simulink model "CassieRealTimeSubsystem"  (R2016b)
settings: Solver=FixedStepDiscrete  StartTime=0.0  StopTime=inf  RelTol=1e-3  EnableMultiTasking=on
InitFcn:
  | realTimeInitFcn;
undefined symbols (not defined in the file): CassieParameters, leftLegMedulla, pelvisMedulla, rightLegMedulla
libraries: xpcethercatlib x98, RealTimeLibrary x10, slrtlib x4, simulink x3
(part 1 of 2)
settings Model: xpc_rtwmakecfg_data=_xpcethercatlib_  ParamWorkspaceSource=ReferencedWorkspace  Creator=robot  LastModifiedBy=mikha
settings SolverCC: EnableConcurrentExecution=on
settings DataIOCC: SaveFormat=Array  SaveOutput=off  SignalLogging=off  DSMLogging=off  VisualizeSimOutput=off  SaveTime=off
settings OptimizationCC: DefaultParameterBehavior=Inlined  InlineInvariantSignals=on  LifeSpan=inf  SimCompilerOptimization=on  AccelVerboseBuild=on
settings DebuggingCC: AllowSymbolicDim=off  SFUnexpectedBacktrackingDiag=warning  SFNoUnconditionalDefaultTransitionDiag=warning  SFExecutionAtInitializationDiag=none
settings HardwareCC: ProdBitPerPointer=32  ProdBitPerSizeT=32  ProdBitPerPtrDiffT=32  ProdLargestAtomicFloat=None  ProdWordSize=32  ProdLongLongMode=on  ProdHWDeviceType=Generic->32-bit x86 compatible
settings ModelReferenceCC: ParallelModelReferenceMATLABWorkerInit=Copy Base Workspace  ModelReferenceNumInstancesAllowed=Single
settings SFSimCC: SFSimEcho=off
settings RTWCC: SystemTargetFile=slrt.tlc  TLCOptions=-axPCMaxOverloads=1000000000 -axPCMaxOverloadLen=1000000000  TemplateMakefile=slrt_default_tmf  Description=Simulink Real-Time  RTWCompilerOptimization=on
settings CodeAppCC: GenerateComments=off  MaxIdLength=128  SimulinkBlockComments=off
settings SimulinkRealTimeCC: ExtMode=off
settings ConfigComp: CovMetricSettings=dw  CovHtmlReporting=on  CovSaveCumulativeToWorkspaceVar=on  CovSaveSingleToWorkspaceVar=on  CovExternalEMLEnable=off

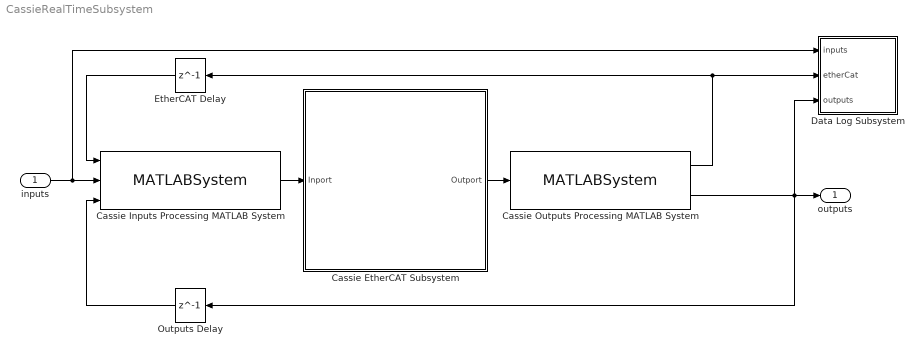
== system CassieRealTimeSubsystem ==
  inputs : Inport  OutDataTypeStr=Bus: cassieInputsBus  PortDimensions=[1 1]  SampleTime=CassieParameters.etherCatSampleTime  BusOutputAsStruct=on
  Cassie EtherCAT Subsystem : Subsystem
      mask Display: image('Cassie.png');
  Cassie Inputs Processing MATLAB System : MATLABSystem  System=ProcessInputs  SimulateUsing=Code generation
      mask Type: ProcessInputs
      mask Display:
      | disp('ProcessInputs');
      | port_label('input',1,'etherCat');
      | port_label('input',2,'inputs');
      | port_label('input',3,'outputs');
      | port_label('output',1,'etherCat');
  Cassie Outputs Processing MATLAB System : MATLABSystem  System=ProcessOutputs  SimulateUsing=Code generation
      mask Type: ProcessOutputs
      mask Display:
      | disp('ProcessOutputs');
      | port_label('input',1,'etherCat');
      | port_label('output',1,'etherCat');
      | port_label('output',2,'outputs');
  Data Log Subsystem : Subsystem
  EtherCAT Delay : Delay  DelayLength=1  InputProcessing=Inherited
  Outputs Delay : Delay  DelayLength=1  InputProcessing=Inherited
  outputs : Outport  OutDataTypeStr=Bus: cassieOutputsBus  PortDimensions=[1 1]  SampleTime=CassieParameters.etherCatSampleTime  BusOutputAsStruct=on
  wires:
  inputs/1 -> Data Log Subsystem/1(inputs), Cassie Inputs Processing MATLAB System/2
  Cassie Outputs Processing MATLAB System/2 -> Data Log Subsystem/3(outputs), Outputs Delay/1, outputs/1
  Cassie EtherCAT Subsystem/1(Outport) -> Cassie Outputs Processing MATLAB System/1
  Cassie Outputs Processing MATLAB System/1 -> EtherCAT Delay/1, Data Log Subsystem/2(etherCat)
  Cassie Inputs Processing MATLAB System/1 -> Cassie EtherCAT Subsystem/1(Inport)
  EtherCAT Delay/1 -> Cassie Inputs Processing MATLAB System/1
  Outputs Delay/1 -> Cassie Inputs Processing MATLAB System/3

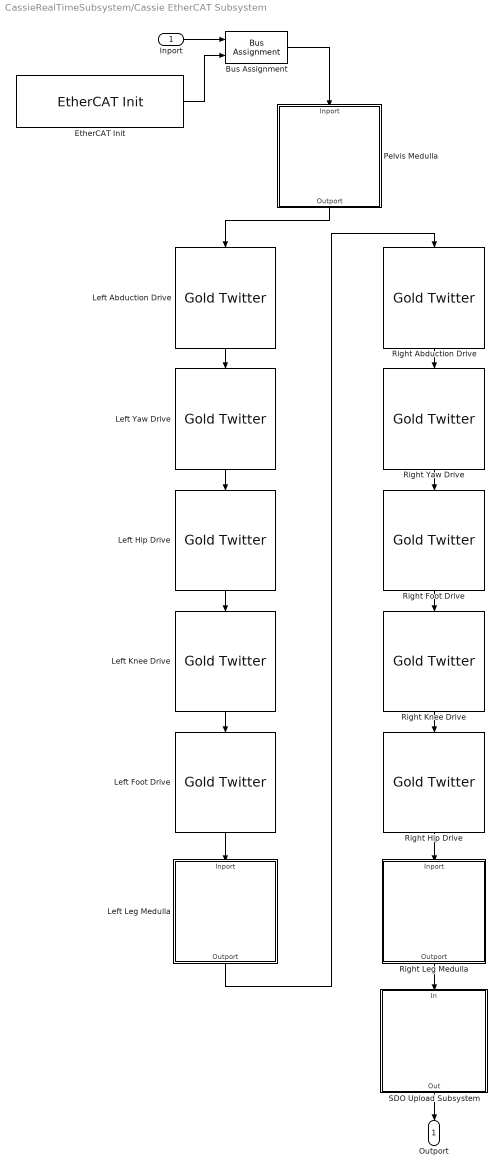
== system CassieRealTimeSubsystem/Cassie EtherCAT Subsystem ==
  Inport : Inport
  Bus Assignment : BusAssignment  AssignedSignals=status
  "EtherCAT Init " : xpcethercatlib/EtherCAT Init   Priority=0  config_file=cassie-v3-eni.xml  device_id=0  pci_bus=CassieParameters.etherCatPciBus  pci_slot=CassieParameters.etherCatPciSlot  dctuning=0  enaDebug=off  enaDC=on  errLink=on  masterDbg=on  stateChgDbg=on  baseClock=on  masterCfg=on  logFile='c:\dbglog2.txt'  sample_time=0.000500  DCMode=1
  Left Abduction Drive : RealTimeLibrary/Gold Twitter  structureName='leftAbductionDrive'  ethercatName='Left Abduction Drive'  gearRatio=CassieParameters.motorGearRatio(1)*CassieParameters.motorDirection(1)  torqueConstant=CassieParameters.motorTorqueConstant(1)  encoderCounts=CassieParameters.motorEncoderTicks(1)  peakCurrentLimit=CassieParameters.twitterPeakCurrent(1)
  Left Foot Drive : RealTimeLibrary/Gold Twitter  structureName='leftFootDrive'  ethercatName='Left Foot Drive'  gearRatio=CassieParameters.motorGearRatio(5)*CassieParameters.motorDirection(5)  torqueConstant=CassieParameters.motorTorqueConstant(5)  encoderCounts=CassieParameters.motorEncoderTicks(5)  peakCurrentLimit=CassieParameters.twitterPeakCurrent(5)
  Left Hip Drive : RealTimeLibrary/Gold Twitter  structureName='leftHipDrive'  ethercatName='Left Hip Drive'  gearRatio=CassieParameters.motorGearRatio(3)*CassieParameters.motorDirection(3)  torqueConstant=CassieParameters.motorTorqueConstant(3)  encoderCounts=CassieParameters.motorEncoderTicks(3)  peakCurrentLimit=CassieParameters.twitterPeakCurrent(3)
  Left Knee Drive : RealTimeLibrary/Gold Twitter  structureName='leftKneeDrive'  ethercatName='Left Knee Drive'  gearRatio=CassieParameters.motorGearRatio(4)*CassieParameters.motorDirection(4)  torqueConstant=CassieParameters.motorTorqueConstant(4)  encoderCounts=CassieParameters.motorEncoderTicks(4)  peakCurrentLimit=CassieParameters.twitterPeakCurrent(4)
  Left Leg Medulla : Subsystem
      mask Display: image('Medulla.png');
  Left Yaw Drive : RealTimeLibrary/Gold Twitter  structureName='leftYawDrive'  ethercatName='Left Yaw Drive'  gearRatio=CassieParameters.motorGearRatio(2)*CassieParameters.motorDirection(2)  torqueConstant=CassieParameters.motorTorqueConstant(2)  encoderCounts=CassieParameters.motorEncoderTicks(2)  peakCurrentLimit=CassieParameters.twitterPeakCurrent(2)
  Pelvis Medulla : Subsystem
      mask Display: image('Medulla.png');
  Right Abduction Drive : RealTimeLibrary/Gold Twitter  structureName='rightAbductionDrive'  ethercatName='Right Abduction Drive'  gearRatio=CassieParameters.motorGearRatio(6)*CassieParameters.motorDirection(6)  torqueConstant=CassieParameters.motorTorqueConstant(6)  encoderCounts=CassieParameters.motorEncoderTicks(6)  peakCurrentLimit=CassieParameters.twitterPeakCurrent(6)
  Right Foot Drive : RealTimeLibrary/Gold Twitter  structureName='rightFootDrive'  ethercatName='Right Foot Drive'  gearRatio=CassieParameters.motorGearRatio(10)*CassieParameters.motorDirection(10)  torqueConstant=CassieParameters.motorTorqueConstant(10)  encoderCounts=CassieParameters.motorEncoderTicks(10)  peakCurrentLimit=CassieParameters.twitterPeakCurrent(10)
  Right Hip Drive : RealTimeLibrary/Gold Twitter  structureName='rightHipDrive'  ethercatName='Right Hip Drive'  gearRatio=CassieParameters.motorGearRatio(8)*CassieParameters.motorDirection(8)  torqueConstant=CassieParameters.motorTorqueConstant(8)  encoderCounts=CassieParameters.motorEncoderTicks(8)  peakCurrentLimit=CassieParameters.twitterPeakCurrent(8)
  Right Knee Drive : RealTimeLibrary/Gold Twitter  structureName='rightKneeDrive'  ethercatName='Right Knee Drive'  gearRatio=CassieParameters.motorGearRatio(9)*CassieParameters.motorDirection(9)  torqueConstant=CassieParameters.motorTorqueConstant(9)  encoderCounts=CassieParameters.motorEncoderTicks(9)  peakCurrentLimit=CassieParameters.twitterPeakCurrent(9)
  Right Leg Medulla : Subsystem
      mask Display: image('Medulla.png');
  Right Yaw Drive : RealTimeLibrary/Gold Twitter  structureName='rightYawDrive'  ethercatName='Right Yaw Drive'  gearRatio=CassieParameters.motorGearRatio(7)*CassieParameters.motorDirection(7)  torqueConstant=CassieParameters.motorTorqueConstant(7)  encoderCounts=CassieParameters.motorEncoderTicks(7)  peakCurrentLimit=CassieParameters.twitterPeakCurrent(7)
  SDO Upload Subsystem : Subsystem
  Outport : Outport
  wires:
  Bus Assignment/1 -> Pelvis Medulla/1(Inport)
  SDO Upload Subsystem/1(Out) -> Outport/1
  Right Leg Medulla/1(Outport) -> SDO Upload Subsystem/1(In)
  Right Abduction Drive/1 -> Right Yaw Drive/1
  Left Leg Medulla/1(Outport) -> Right Abduction Drive/1
  Left Knee Drive/1 -> Left Foot Drive/1
  Left Hip Drive/1 -> Left Knee Drive/1
  Left Yaw Drive/1 -> Left Hip Drive/1
  Left Abduction Drive/1 -> Left Yaw Drive/1
  Inport/1 -> Bus Assignment/1
  "EtherCAT Init "/1 -> Bus Assignment/2
  Left Foot Drive/1 -> Left Leg Medulla/1(Inport)
  Right Knee Drive/1 -> Right Hip Drive/1
  Right Yaw Drive/1 -> Right Foot Drive/1
  Right Foot Drive/1 -> Right Knee Drive/1
  Right Hip Drive/1 -> Right Leg Medulla/1(Inport)
  Pelvis Medulla/1(Outport) -> Left Abduction Drive/1

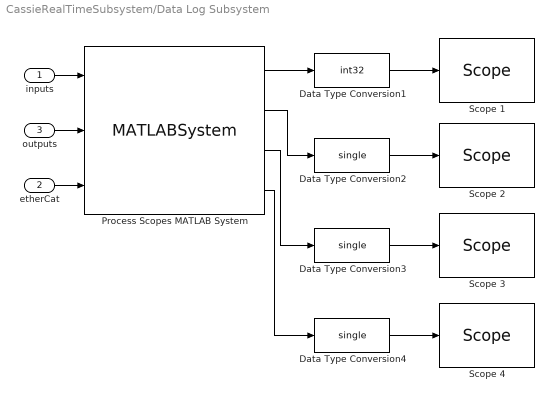
== system CassieRealTimeSubsystem/Data Log Subsystem ==
  inputs : Inport  OutDataTypeStr=Bus: cassieInputsBus
  etherCat : Inport  Port=2  OutDataTypeStr=Bus: cassieEtherCatBus
  outputs : Inport  Port=3  OutDataTypeStr=Bus: cassieOutputsBus
  Data Type Conversion1 : DataTypeConversion  OutDataTypeStr=int32
  Data Type Conversion2 : DataTypeConversion  OutDataTypeStr=single
  Data Type Conversion3 : DataTypeConversion  OutDataTypeStr=single
  Data Type Conversion4 : DataTypeConversion  OutDataTypeStr=single
  Process Scopes MATLAB System : MATLABSystem  System=ProcessScopes  SimulateUsing=Code generation
      mask Type: ProcessScopes
      mask Display:
      | disp('ProcessScopes');
      | port_label('input',1,'inputs');
      | port_label('input',2,'outputs');
      | port_label('input',3,'etherCat');
      | port_label('output',1,'messageLog');
      | port_label('output',2,'energyLog');
      | port_label('output',3,'inputsLog');
      | port_label('output',4,'outputsLog');
  Scope 1 : slrtlib/Displays and Logging/Scope   scopeno=1  scopetype=File  autostart=on  viewmode=Graphical redraw  formatstr='%15.6f'  grid=on  ylimits=[0,0]  nosamples=250  noprepostsamples=0  interleave=1  triggermode=FreeRun  triggersignal=1  trigsignalfromport=on  triggerlevel=2  triggerslope=Rising  triggerscope=1  triggersample=0  filename=message.dat  mode=Commit  writesize=512  autorestart=on  dynamicfilemode=off  maxwritefilesize=4000*1024^2
  Scope 2 : slrtlib/Displays and Logging/Scope   scopeno=2  scopetype=File  autostart=on  viewmode=Graphical redraw  formatstr='%15.6f'  grid=on  ylimits=[0,0]  nosamples=250  noprepostsamples=0  interleave=1  triggermode=FreeRun  triggersignal=1  trigsignalfromport=on  triggerlevel=0.5  triggerslope=Rising  triggerscope=1  triggersample=0  filename=energy.dat  mode=Commit  writesize=512  autorestart=on  dynamicfilemode=off  maxwritefilesize=4000*1024^2
  Scope 3 : slrtlib/Displays and Logging/Scope   scopeno=3  scopetype=File  autostart=on  viewmode=Numerical  formatstr='%15.6f'  grid=on  ylimits=[0,0]  nosamples=250  noprepostsamples=0  interleave=1  triggermode=FreeRun  triggersignal=1  trigsignalfromport=on  triggerlevel=0.5  triggerslope=Rising  triggerscope=1  triggersample=0  filename=inputs.dat  mode=Commit  writesize=512  autorestart=on  dynamicfilemode=off  maxwritefilesize=4000*1024^2
  Scope 4 : slrtlib/Displays and Logging/Scope   scopeno=4  scopetype=File  autostart=on  viewmode=Numerical  formatstr='%15.6f'  grid=on  ylimits=[0,0]  nosamples=250  noprepostsamples=0  interleave=1  triggermode=FreeRun  triggersignal=1  trigsignalfromport=on  triggerlevel=0.5  triggerslope=Rising  triggerscope=1  triggersample=0  filename=outputs.dat  mode=Commit  writesize=512  autorestart=on  dynamicfilemode=off  maxwritefilesize=4000*1024^2
  wires:
  Process Scopes MATLAB System/4 -> Data Type Conversion4/1
  Process Scopes MATLAB System/3 -> Data Type Conversion3/1
  Process Scopes MATLAB System/2 -> Data Type Conversion2/1
  Process Scopes MATLAB System/1 -> Data Type Conversion1/1
  outputs/1 -> Process Scopes MATLAB System/2
  etherCat/1 -> Process Scopes MATLAB System/3
  inputs/1 -> Process Scopes MATLAB System/1
  Data Type Conversion1/1 -> Scope 1/1
  Data Type Conversion2/1 -> Scope 2/1
  Data Type Conversion3/1 -> Scope 3/1
  Data Type Conversion4/1 -> Scope 4/1

== system CassieRealTimeSubsystem/Cassie EtherCAT Subsystem/Left Leg Medulla ==
  Inport : Inport
  Base Medulla : Subsystem  mask{structureName='leftLegMedulla', ethercatName='Left Leg Medulla'}
      mask prompts: structureName "Structure Name"; ethercatName "EtherCAT Name"
      mask init:
      | % Set bus assignments
      | set_param([gcb '/Base Inputs Bus Assignment'], ...
      |   'AssignedSignals', [...
      |     structureName '.baseInputs.cpuLoad,', ...
      |     structureName '.baseInputs.counter']);
      | 
      | % Set PDO recieve signal names
      | set_param([gcb '/CPU Load PDO Receive'], ...
      |   'sig_name', [ethercatName '.Base Inputs.CPU Load']);
      | set_param([gcb '/Counter PDO Receive'], ...
      |   'sig_name', [ethercatName '.Base Inputs.Counter']);
      mask Display: image('Medulla.png');
  Misc Inputs : Subsystem
  Outport : Outport  LockScale=on
  wires:
  Misc Inputs/1(Outport) -> Outport/1
  Inport/1 -> Base Medulla/1(Inport)
  Base Medulla/1(Outport) -> Misc Inputs/1(Inport)

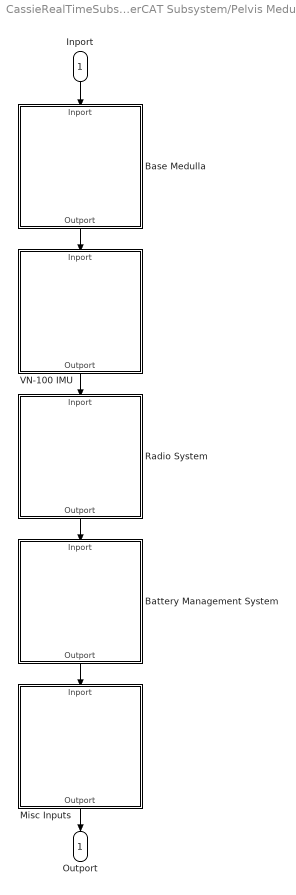
== system CassieRealTimeSubsystem/Cassie EtherCAT Subsystem/Pelvis Medulla ==
  Inport : Inport
  Base Medulla : Subsystem  mask{structureName='pelvisMedulla', ethercatName='Pelvis Medulla'}
      mask prompts: structureName "Structure Name"; ethercatName "EtherCAT Name"
      mask init: same as CassieRealTimeSubsystem/Cassie EtherCAT Subsystem/Left Leg Medulla/Base Medulla
      mask Display: image('Medulla.png');
  Battery Management System : Subsystem
      mask Display: image('BQ76PL536A.png');
  Misc Inputs : Subsystem
  Radio System : Subsystem
      mask Display: image('Fr Sky Taranis.png');
  VN-100 IMU : Subsystem
      mask Display: image('VN-100 IMU.png');
  Outport : Outport
  wires:
  VN-100 IMU/1(Outport) -> Radio System/1(Inport)
  Radio System/1(Outport) -> Battery Management System/1(Inport)
  Misc Inputs/1(Outport) -> Outport/1
  Inport/1 -> Base Medulla/1(Inport)
  Battery Management System/1(Outport) -> Misc Inputs/1(Inport)
  Base Medulla/1(Outport) -> VN-100 IMU/1(Inport)

== system CassieRealTimeSubsystem/Cassie EtherCAT Subsystem/Right Leg Medulla ==
  Inport : Inport
  Base Medulla : Subsystem  mask{structureName='rightLegMedulla', ethercatName='Right Leg Medulla'}
      mask prompts: structureName "Structure Name"; ethercatName "EtherCAT Name"
      mask init: same as CassieRealTimeSubsystem/Cassie EtherCAT Subsystem/Left Leg Medulla/Base Medulla
      mask Display: image('Medulla.png');
  Misc Inputs : Subsystem
  Outport : Outport
  wires:
  Inport/1 -> Base Medulla/1(Inport)
  Base Medulla/1(Outport) -> Misc Inputs/1(Inport)
  Misc Inputs/1(Outport) -> Outport/1

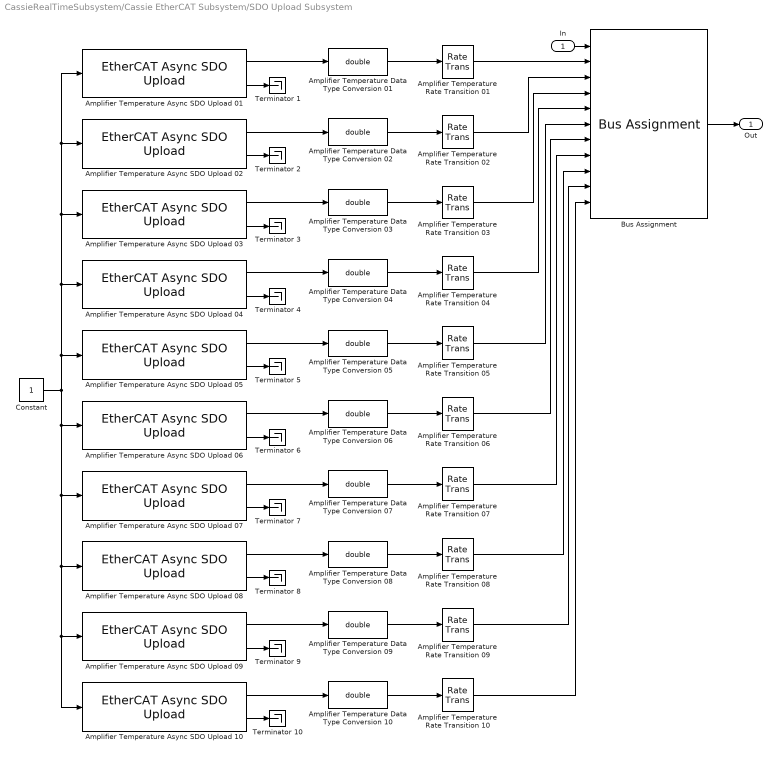
== system CassieRealTimeSubsystem/Cassie EtherCAT Subsystem/SDO Upload Subsystem ==
  In : Inport
  Amplifier Temperature Data Type Conversion 01 : DataTypeConversion  OutDataTypeStr=double
  Amplifier Temperature Data Type Conversion 02 : DataTypeConversion  OutDataTypeStr=double
  Amplifier Temperature Data Type Conversion 03 : DataTypeConversion  OutDataTypeStr=double
  Amplifier Temperature Data Type Conversion 04 : DataTypeConversion  OutDataTypeStr=double
  Amplifier Temperature Data Type Conversion 05 : DataTypeConversion  OutDataTypeStr=double
  Amplifier Temperature Data Type Conversion 06 : DataTypeConversion  OutDataTypeStr=double
  Amplifier Temperature Data Type Conversion 07 : DataTypeConversion  OutDataTypeStr=double
  Amplifier Temperature Data Type Conversion 08 : DataTypeConversion  OutDataTypeStr=double
  Amplifier Temperature Data Type Conversion 09 : DataTypeConversion  OutDataTypeStr=double
  Amplifier Temperature Data Type Conversion 10 : DataTypeConversion  OutDataTypeStr=double
  Amplifier Temperature Rate Transition 01 : RateTransition  Deterministic=off
  Amplifier Temperature Rate Transition 02 : RateTransition  Deterministic=off
  Amplifier Temperature Rate Transition 03 : RateTransition  Deterministic=off
  Amplifier Temperature Rate Transition 04 : RateTransition  Deterministic=off
  Amplifier Temperature Rate Transition 05 : RateTransition  Deterministic=off
  Amplifier Temperature Rate Transition 06 : RateTransition  Deterministic=off
  Amplifier Temperature Rate Transition 07 : RateTransition  Deterministic=off
  Amplifier Temperature Rate Transition 08 : RateTransition  Deterministic=off
  Amplifier Temperature Rate Transition 09 : RateTransition  Deterministic=off
  Amplifier Temperature Rate Transition 10 : RateTransition  Deterministic=off
  Amplifier Temperature Async SDO Upload 01 : xpcethercatlib/EtherCAT Async SDO Upload  index=8867  subIndex=1  sig_type=int16  sig_dim=1  device_id=0  slave_name=Left Abduction Drive  sample_time=1  slave_addr=1002  selected_slave=Term 1 (EK1100)  timeout=500  slave_found=1
  Amplifier Temperature Async SDO Upload 02 : xpcethercatlib/EtherCAT Async SDO Upload  index=8867  subIndex=1  sig_type=int16  sig_dim=1  device_id=0  slave_name=Left Yaw Drive  sample_time=1  slave_addr=1003  selected_slave=Term 1 (EK1100)  timeout=500  slave_found=1
  Amplifier Temperature Async SDO Upload 03 : xpcethercatlib/EtherCAT Async SDO Upload  index=8867  subIndex=1  sig_type=int16  sig_dim=1  device_id=0  slave_name=Left Hip Drive  sample_time=1  slave_addr=1004  selected_slave=Term 1 (EK1100)  timeout=500  slave_found=1
  Amplifier Temperature Async SDO Upload 04 : xpcethercatlib/EtherCAT Async SDO Upload  index=8867  subIndex=1  sig_type=int16  sig_dim=1  device_id=0  slave_name=Left Knee Drive  sample_time=1  slave_addr=1005  selected_slave=Term 1 (EK1100)  timeout=500  slave_found=1
  Amplifier Temperature Async SDO Upload 05 : xpcethercatlib/EtherCAT Async SDO Upload  index=8867  subIndex=1  sig_type=int16  sig_dim=1  device_id=0  slave_name=Left Foot Drive  sample_time=1  slave_addr=1006  selected_slave=Term 1 (EK1100)  timeout=500  slave_found=1
  Amplifier Temperature Async SDO Upload 06 : xpcethercatlib/EtherCAT Async SDO Upload  index=8867  subIndex=1  sig_type=int16  sig_dim=1  device_id=0  slave_name=Right Abduction Drive  sample_time=1  slave_addr=1008  selected_slave=Term 1 (EK1100)  timeout=500  slave_found=1
  Amplifier Temperature Async SDO Upload 07 : xpcethercatlib/EtherCAT Async SDO Upload  index=8867  subIndex=1  sig_type=int16  sig_dim=1  device_id=0  slave_name=Right Yaw Drive  sample_time=1  slave_addr=1009  selected_slave=Term 1 (EK1100)  timeout=500  slave_found=1
  Amplifier Temperature Async SDO Upload 08 : xpcethercatlib/EtherCAT Async SDO Upload  index=8867  subIndex=1  sig_type=int16  sig_dim=1  device_id=0  slave_name=Right Hip Drive  sample_time=1  slave_addr=1012  selected_slave=Term 1 (EK1100)  timeout=500  slave_found=1
  Amplifier Temperature Async SDO Upload 09 : xpcethercatlib/EtherCAT Async SDO Upload  index=8867  subIndex=1  sig_type=int16  sig_dim=1  device_id=0  slave_name=Right Knee Drive  sample_time=1  slave_addr=1011  selected_slave=Term 1 (EK1100)  timeout=500  slave_found=1
  Amplifier Temperature Async SDO Upload 10 : xpcethercatlib/EtherCAT Async SDO Upload  index=8867  subIndex=1  sig_type=int16  sig_dim=1  device_id=0  slave_name=Right Foot Drive  sample_time=1  slave_addr=1010  selected_slave=Term 1 (EK1100)  timeout=500  slave_found=1
  Bus Assignment : BusAssignment  AssignedSignals=leftAbductionDrive.inputs.amplifierTemperature,leftYawDrive.inputs.amplifierTemperature,leftHipDrive.inputs.amplifierTemperature,leftKneeDrive.inputs.amplifierTemperature,leftFootDrive.inputs.amplifierTemperature,rightAbductionDrive.inputs.amplifierTemperature,rightYawDrive.inputs.amplifierTemperature,rightHipDrive.inputs.amplifierTemperature,rightKneeDrive.inputs.amplifierTemperature,rightFootDrive.inputs.amplifierTemperature
  Constant : Constant  OutDataTypeStr=int32
  Terminator {1..10} (10 alike) : Terminator
  Out : Outport
  wires:
  Amplifier Temperature Async SDO Upload 10/2 -> Terminator 10/1
  Amplifier Temperature Async SDO Upload 09/2 -> Terminator 9/1
  Amplifier Temperature Async SDO Upload 08/2 -> Terminator 8/1
  Amplifier Temperature Async SDO Upload 07/2 -> Terminator 7/1
  Amplifier Temperature Async SDO Upload 06/2 -> Terminator 6/1
  Amplifier Temperature Async SDO Upload 05/2 -> Terminator 5/1
  Amplifier Temperature Async SDO Upload 04/2 -> Terminator 4/1
  Amplifier Temperature Async SDO Upload 02/2 -> Terminator 2/1
  Amplifier Temperature Async SDO Upload 03/2 -> Terminator 3/1
  Amplifier Temperature Async SDO Upload 01/2 -> Terminator 1/1
  Amplifier Temperature Rate Transition 10/1 -> Bus Assignment/11
  Amplifier Temperature Rate Transition 09/1 -> Bus Assignment/10
  Amplifier Temperature Rate Transition 08/1 -> Bus Assignment/9
  Amplifier Temperature Rate Transition 07/1 -> Bus Assignment/8
  Amplifier Temperature Rate Transition 06/1 -> Bus Assignment/7
  Amplifier Temperature Rate Transition 05/1 -> Bus Assignment/6
  Amplifier Temperature Rate Transition 04/1 -> Bus Assignment/5
  Amplifier Temperature Rate Transition 03/1 -> Bus Assignment/4
  Amplifier Temperature Rate Transition 02/1 -> Bus Assignment/3
  Amplifier Temperature Data Type Conversion 10/1 -> Amplifier Temperature Rate Transition 10/1
  Amplifier Temperature Data Type Conversion 09/1 -> Amplifier Temperature Rate Transition 09/1
  Amplifier Temperature Data Type Conversion 08/1 -> Amplifier Temperature Rate Transition 08/1
  Amplifier Temperature Data Type Conversion 07/1 -> Amplifier Temperature Rate Transition 07/1
  Amplifier Temperature Data Type Conversion 06/1 -> Amplifier Temperature Rate Transition 06/1
  Amplifier Temperature Data Type Conversion 05/1 -> Amplifier Temperature Rate Transition 05/1
  Amplifier Temperature Data Type Conversion 04/1 -> Amplifier Temperature Rate Transition 04/1
  Amplifier Temperature Data Type Conversion 03/1 -> Amplifier Temperature Rate Transition 03/1
  Amplifier Temperature Data Type Conversion 02/1 -> Amplifier Temperature Rate Transition 02/1
  Constant/1 -> Amplifier Temperature Async SDO Upload 05/1, Amplifier Temperature Async SDO Upload 04/1, Amplifier Temperature Async SDO Upload 03/1, Amplifier Temperature Async SDO Upload 02/1, Amplifier Temperature Async SDO Upload 01/1, Amplifier Temperature Async SDO Upload 06/1, Amplifier Temperature Async SDO Upload 07/1, Amplifier Temperature Async SDO Upload 08/1, Amplifier Temperature Async SDO Upload 09/1, Amplifier Temperature Async SDO Upload 10/1
  Amplifier Temperature Async SDO Upload 08/1 -> Amplifier Temperature Data Type Conversion 08/1
  In/1 -> Bus Assignment/1
  Bus Assignment/1 -> Out/1
  Amplifier Temperature Async SDO Upload 05/1 -> Amplifier Temperature Data Type Conversion 05/1
  Amplifier Temperature Async SDO Upload 01/1 -> Amplifier Temperature Data Type Conversion 01/1
  Amplifier Temperature Rate Transition 01/1 -> Bus Assignment/2
  Amplifier Temperature Data Type Conversion 01/1 -> Amplifier Temperature Rate Transition 01/1
  Amplifier Temperature Async SDO Upload 06/1 -> Amplifier Temperature Data Type Conversion 06/1
  Amplifier Temperature Async SDO Upload 04/1 -> Amplifier Temperature Data Type Conversion 04/1
  Amplifier Temperature Async SDO Upload 03/1 -> Amplifier Temperature Data Type Conversion 03/1
  Amplifier Temperature Async SDO Upload 09/1 -> Amplifier Temperature Data Type Conversion 09/1
  Amplifier Temperature Async SDO Upload 07/1 -> Amplifier Temperature Data Type Conversion 07/1
  Amplifier Temperature Async SDO Upload 10/1 -> Amplifier Temperature Data Type Conversion 10/1
  Amplifier Temperature Async SDO Upload 02/1 -> Amplifier Temperature Data Type Conversion 02/1

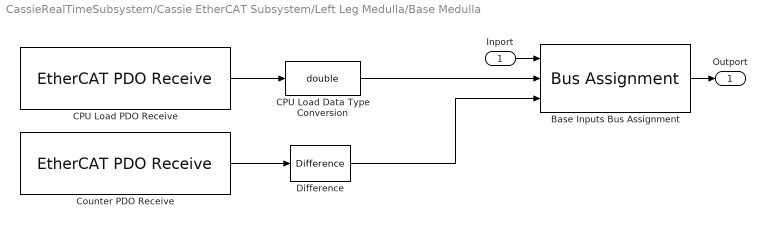
== system CassieRealTimeSubsystem/Cassie EtherCAT Subsystem/Left Leg Medulla/Base Medulla ==
  Inport : Inport
  Base Inputs Bus Assignment : BusAssignment  AssignedSignals=leftLegMedulla.baseInputs.cpuLoad,leftLegMedulla.baseInputs.counter
  CPU Load Data Type Conversion : DataTypeConversion  OutDataTypeStr=double
  CPU Load PDO Receive : xpcethercatlib/EtherCAT PDO Receive  Priority=2  sig_name=Left Leg Medulla.Base Inputs.CPU Load  sig_offset=1856  sig_type=uint16  type_size=16  sig_dim=1  device_id=0  sample_time=0.000500
  Counter PDO Receive : xpcethercatlib/EtherCAT PDO Receive  Priority=2  sig_name=Left Leg Medulla.Base Inputs.Counter  sig_offset=1848  sig_type=uint8  type_size=8  sig_dim=1  device_id=0  sample_time=0.000500
  Difference : simulink/Discrete/Difference  ICPrevInput=0.0  OutMin=[]  OutMax=[]  OutDataType=fixdt(1, 16)  OutScaling=2^-10  DoSatur=off
  Outport : Outport
  wires:
  Base Inputs Bus Assignment/1 -> Outport/1
  Counter PDO Receive/1 -> Difference/1
  Difference/1 -> Base Inputs Bus Assignment/3
  Inport/1 -> Base Inputs Bus Assignment/1
  CPU Load PDO Receive/1 -> CPU Load Data Type Conversion/1
  CPU Load Data Type Conversion/1 -> Base Inputs Bus Assignment/2

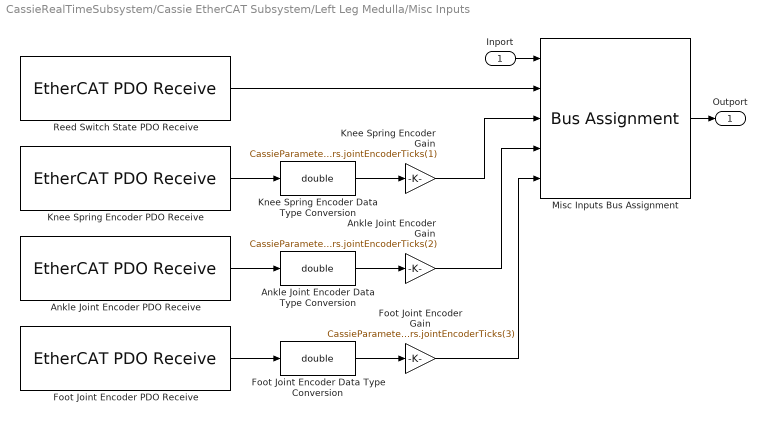
== system CassieRealTimeSubsystem/Cassie EtherCAT Subsystem/Left Leg Medulla/Misc Inputs ==
  Inport : Inport
  Ankle Joint Encoder Data Type Conversion : DataTypeConversion  OutDataTypeStr=double
  Ankle Joint Encoder Gain : Gain  Gain=CassieParameters.jointDirection(2)*2*pi/CassieParameters.jointEncoderTicks(2)
  Ankle Joint Encoder PDO Receive : xpcethercatlib/EtherCAT PDO Receive  Priority=2  sig_name=Left Leg Medulla.Misc Inputs.Ankle Joint Encoder  sig_offset=1904  sig_type=int32  type_size=32  sig_dim=1  device_id=0  sample_time=0.000500
  Foot Joint Encoder Data Type Conversion : DataTypeConversion  OutDataTypeStr=double
  Foot Joint Encoder Gain : Gain  Gain=CassieParameters.jointDirection(3)*2*pi/CassieParameters.jointEncoderTicks(3)
  Foot Joint Encoder PDO Receive : xpcethercatlib/EtherCAT PDO Receive  Priority=2  sig_name=Left Leg Medulla.Misc Inputs.Foot Joint Encoder  sig_offset=1936  sig_type=int32  type_size=32  sig_dim=1  device_id=0  sample_time=0.000500
  Knee Spring Encoder Data Type Conversion : DataTypeConversion  OutDataTypeStr=double
  Knee Spring Encoder Gain : Gain  Gain=CassieParameters.jointDirection(1)*2*pi/CassieParameters.jointEncoderTicks(1)
  Knee Spring Encoder PDO Receive : xpcethercatlib/EtherCAT PDO Receive  Priority=2  sig_name=Left Leg Medulla.Misc Inputs.Knee Spring Encoder  sig_offset=1872  sig_type=int32  type_size=32  sig_dim=1  device_id=0  sample_time=0.000500
  Misc Inputs Bus Assignment : BusAssignment  AssignedSignals=leftLegMedulla.miscInputs.reedSwitchState,leftLegMedulla.miscInputs.kneeSpringEncoder,leftLegMedulla.miscInputs.ankleJointEncoder,leftLegMedulla.miscInputs.footJointEncoder
  Reed Switch State PDO Receive : xpcethercatlib/EtherCAT PDO Receive  Priority=2  sig_name=Left Leg Medulla.Misc Inputs.Reed Switch  sig_offset=1968  sig_type=boolean  type_size=1  sig_dim=1  device_id=0  sample_time=0.000500
  Outport : Outport  LockScale=on
  wires:
  Reed Switch State PDO Receive/1 -> Misc Inputs Bus Assignment/2
  Ankle Joint Encoder Data Type Conversion/1 -> Ankle Joint Encoder Gain/1
  Knee Spring Encoder Data Type Conversion/1 -> Knee Spring Encoder Gain/1
  Foot Joint Encoder PDO Receive/1 -> Foot Joint Encoder Data Type Conversion/1
  Foot Joint Encoder Data Type Conversion/1 -> Foot Joint Encoder Gain/1
  Misc Inputs Bus Assignment/1 -> Outport/1
  Knee Spring Encoder PDO Receive/1 -> Knee Spring Encoder Data Type Conversion/1
  Ankle Joint Encoder PDO Receive/1 -> Ankle Joint Encoder Data Type Conversion/1
  Inport/1 -> Misc Inputs Bus Assignment/1
  Foot Joint Encoder Gain/1 -> Misc Inputs Bus Assignment/5
  Ankle Joint Encoder Gain/1 -> Misc Inputs Bus Assignment/4
  Knee Spring Encoder Gain/1 -> Misc Inputs Bus Assignment/3

== system CassieRealTimeSubsystem/Cassie EtherCAT Subsystem/Pelvis Medulla/Base Medulla ==
  Inport : Inport
  Base Inputs Bus Assignment : BusAssignment  AssignedSignals=pelvisMedulla.baseInputs.cpuLoad,pelvisMedulla.baseInputs.counter
  CPU Load Data Type Conversion : DataTypeConversion  OutDataTypeStr=double
  CPU Load PDO Receive : xpcethercatlib/EtherCAT PDO Receive  Priority=2  sig_name=Pelvis Medulla.Base Inputs.CPU Load  sig_offset=600  sig_type=uint16  type_size=16  sig_dim=1  device_id=0  sample_time=0.000500
  Counter PDO Receive : xpcethercatlib/EtherCAT PDO Receive  Priority=2  sig_name=Pelvis Medulla.Base Inputs.Counter  sig_offset=592  sig_type=uint8  type_size=8  sig_dim=1  device_id=0  sample_time=0.000500
  Difference : simulink/Discrete/Difference  ICPrevInput=0.0  OutMin=[]  OutMax=[]  OutDataType=fixdt(1, 16)  OutScaling=2^-10  DoSatur=off
  Outport : Outport
  wires:
  Base Inputs Bus Assignment/1 -> Outport/1
  Counter PDO Receive/1 -> Difference/1
  Difference/1 -> Base Inputs Bus Assignment/3
  Inport/1 -> Base Inputs Bus Assignment/1
  CPU Load PDO Receive/1 -> CPU Load Data Type Conversion/1
  CPU Load Data Type Conversion/1 -> Base Inputs Bus Assignment/2

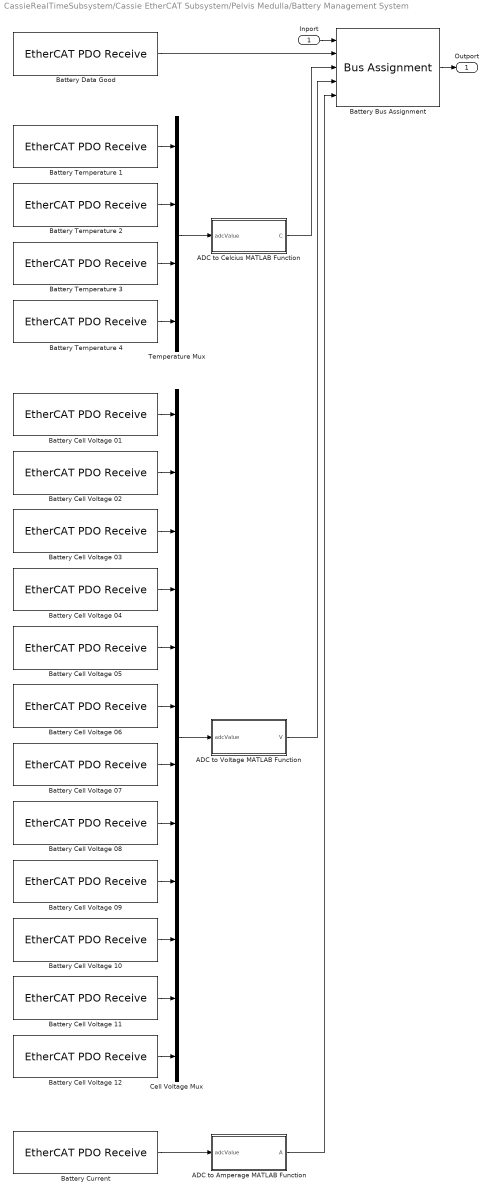
== system CassieRealTimeSubsystem/Cassie EtherCAT Subsystem/Pelvis Medulla/Battery Management System ==
  Inport : Inport
  ADC to Amperage MATLAB Function : MATLAB Function  TreatAsAtomicUnit=on
  ADC to Celcius MATLAB Function : MATLAB Function  TreatAsAtomicUnit=on
  ADC to Voltage MATLAB Function : MATLAB Function  TreatAsAtomicUnit=on
  Battery Bus Assignment : BusAssignment  AssignedSignals=pelvisMedulla.bmsInputs.dataGood,pelvisMedulla.bmsInputs.temperature,pelvisMedulla.bmsInputs.cellVoltage,pelvisMedulla.bmsInputs.current
  Battery Cell Voltage 01 : xpcethercatlib/EtherCAT PDO Receive  Priority=2  sig_name=Pelvis Medulla.BMS Inputs.Cell Voltage 01  sig_offset=1544  sig_type=uint16  type_size=16  sig_dim=1  device_id=0  sample_time=0.000500
  Battery Cell Voltage 02 : xpcethercatlib/EtherCAT PDO Receive  Priority=2  sig_name=Pelvis Medulla.BMS Inputs.Cell Voltage 02  sig_offset=1560  sig_type=uint16  type_size=16  sig_dim=1  device_id=0  sample_time=0.000500
  Battery Cell Voltage 03 : xpcethercatlib/EtherCAT PDO Receive  Priority=2  sig_name=Pelvis Medulla.BMS Inputs.Cell Voltage 03  sig_offset=1576  sig_type=uint16  type_size=16  sig_dim=1  device_id=0  sample_time=0.000500
  Battery Cell Voltage 04 : xpcethercatlib/EtherCAT PDO Receive  Priority=2  sig_name=Pelvis Medulla.BMS Inputs.Cell Voltage 04  sig_offset=1592  sig_type=uint16  type_size=16  sig_dim=1  device_id=0  sample_time=0.000500
  Battery Cell Voltage 05 : xpcethercatlib/EtherCAT PDO Receive  Priority=2  sig_name=Pelvis Medulla.BMS Inputs.Cell Voltage 05  sig_offset=1608  sig_type=uint16  type_size=16  sig_dim=1  device_id=0  sample_time=0.000500
  Battery Cell Voltage 06 : xpcethercatlib/EtherCAT PDO Receive  Priority=2  sig_name=Pelvis Medulla.BMS Inputs.Cell Voltage 06  sig_offset=1624  sig_type=uint16  type_size=16  sig_dim=1  device_id=0  sample_time=0.000500
  Battery Cell Voltage 07 : xpcethercatlib/EtherCAT PDO Receive  Priority=2  sig_name=Pelvis Medulla.BMS Inputs.Cell Voltage 07  sig_offset=1640  sig_type=uint16  type_size=16  sig_dim=1  device_id=0  sample_time=0.000500
  Battery Cell Voltage 08 : xpcethercatlib/EtherCAT PDO Receive  Priority=2  sig_name=Pelvis Medulla.BMS Inputs.Cell Voltage 08  sig_offset=1656  sig_type=uint16  type_size=16  sig_dim=1  device_id=0  sample_time=0.000500
  Battery Cell Voltage 09 : xpcethercatlib/EtherCAT PDO Receive  Priority=2  sig_name=Pelvis Medulla.BMS Inputs.Cell Voltage 09  sig_offset=1672  sig_type=uint16  type_size=16  sig_dim=1  device_id=0  sample_time=0.000500
  Battery Cell Voltage 10 : xpcethercatlib/EtherCAT PDO Receive  Priority=2  sig_name=Pelvis Medulla.BMS Inputs.Cell Voltage 10  sig_offset=1688  sig_type=uint16  type_size=16  sig_dim=1  device_id=0  sample_time=0.000500
  Battery Cell Voltage 11 : xpcethercatlib/EtherCAT PDO Receive  Priority=2  sig_name=Pelvis Medulla.BMS Inputs.Cell Voltage 11  sig_offset=1704  sig_type=uint16  type_size=16  sig_dim=1  device_id=0  sample_time=0.000500
  Battery Cell Voltage 12 : xpcethercatlib/EtherCAT PDO Receive  Priority=2  sig_name=Pelvis Medulla.BMS Inputs.Cell Voltage 12  sig_offset=1720  sig_type=uint16  type_size=16  sig_dim=1  device_id=0  sample_time=0.000500
  Battery Current : xpcethercatlib/EtherCAT PDO Receive  Priority=2  sig_name=Pelvis Medulla.BMS Inputs.Current  sig_offset=1800  sig_type=uint16  type_size=16  sig_dim=1  device_id=0  sample_time=0.000500
  Battery Data Good : xpcethercatlib/EtherCAT PDO Receive  Priority=2  sig_name=Pelvis Medulla.BMS Inputs.Data Good  sig_offset=1816  sig_type=boolean  type_size=1  sig_dim=1  device_id=0  sample_time=0.000500
  Battery Temperature 1 : xpcethercatlib/EtherCAT PDO Receive  Priority=2  sig_name=Pelvis Medulla.BMS Inputs.Temperature 1  sig_offset=1736  sig_type=uint16  type_size=16  sig_dim=1  device_id=0  sample_time=0.000500
  Battery Temperature 2 : xpcethercatlib/EtherCAT PDO Receive  Priority=2  sig_name=Pelvis Medulla.BMS Inputs.Temperature 2  sig_offset=1752  sig_type=uint16  type_size=16  sig_dim=1  device_id=0  sample_time=0.000500
  Battery Temperature 3 : xpcethercatlib/EtherCAT PDO Receive  Priority=2  sig_name=Pelvis Medulla.BMS Inputs.Temperature 3  sig_offset=1768  sig_type=uint16  type_size=16  sig_dim=1  device_id=0  sample_time=0.000500
  Battery Temperature 4 : xpcethercatlib/EtherCAT PDO Receive  Priority=2  sig_name=Pelvis Medulla.BMS Inputs.Temperature 4  sig_offset=1784  sig_type=uint16  type_size=16  sig_dim=1  device_id=0  sample_time=0.000500
  Cell Voltage Mux : Mux  Inputs=12
  Temperature Mux : Mux
  Outport : Outport
  wires:
  Battery Temperature 1/1 -> Temperature Mux/1
  Battery Temperature 2/1 -> Temperature Mux/2
  Battery Temperature 3/1 -> Temperature Mux/3
  Battery Temperature 4/1 -> Temperature Mux/4
  Battery Cell Voltage 01/1 -> Cell Voltage Mux/1
  Battery Cell Voltage 02/1 -> Cell Voltage Mux/2
  Battery Cell Voltage 03/1 -> Cell Voltage Mux/3
  Battery Cell Voltage 04/1 -> Cell Voltage Mux/4
  Battery Cell Voltage 05/1 -> Cell Voltage Mux/5
  Battery Cell Voltage 06/1 -> Cell Voltage Mux/6
  Battery Cell Voltage 07/1 -> Cell Voltage Mux/7
  Battery Cell Voltage 08/1 -> Cell Voltage Mux/8
  Battery Cell Voltage 09/1 -> Cell Voltage Mux/9
  Battery Cell Voltage 10/1 -> Cell Voltage Mux/10
  Battery Cell Voltage 11/1 -> Cell Voltage Mux/11
  Battery Cell Voltage 12/1 -> Cell Voltage Mux/12
  ADC to Voltage MATLAB Function/1(V) -> Battery Bus Assignment/4
  ADC to Celcius MATLAB Function/1(C) -> Battery Bus Assignment/3
  Battery Bus Assignment/1 -> Outport/1
  Inport/1 -> Battery Bus Assignment/1
  Temperature Mux/1 -> ADC to Celcius MATLAB Function/1(adcValue)
  Cell Voltage Mux/1 -> ADC to Voltage MATLAB Function/1(adcValue)
  ADC to Amperage MATLAB Function/1(A) -> Battery Bus Assignment/5
  Battery Current/1 -> ADC to Amperage MATLAB Function/1(adcValue)
  Battery Data Good/1 -> Battery Bus Assignment/2

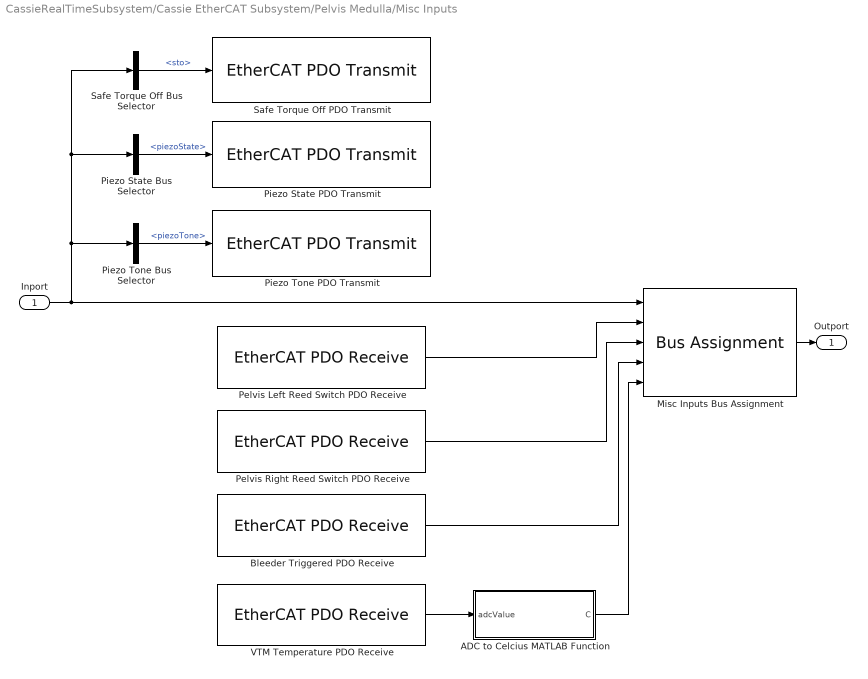
== system CassieRealTimeSubsystem/Cassie EtherCAT Subsystem/Pelvis Medulla/Misc Inputs ==
  Inport : Inport
  ADC to Celcius MATLAB Function : MATLAB Function  TreatAsAtomicUnit=on
  Bleeder Triggered PDO Receive : xpcethercatlib/EtherCAT PDO Receive  Priority=2  sig_name=Pelvis Medulla.Misc Inputs.Bleeder State  sig_offset=1824  sig_type=boolean  type_size=1  sig_dim=1  device_id=0  sample_time=0.000500
  Misc Inputs Bus Assignment : BusAssignment  AssignedSignals=pelvisMedulla.miscInputs.leftReedSwitchState,pelvisMedulla.miscInputs.rightReedSwitchState,pelvisMedulla.miscInputs.bleederState,pelvisMedulla.miscInputs.vtmTemperature
  Pelvis Left Reed Switch PDO Receive : xpcethercatlib/EtherCAT PDO Receive  Priority=2  sig_name=Pelvis Medulla.Misc Inputs.Left Reed Switch State  sig_offset=1826  sig_type=boolean  type_size=1  sig_dim=1  device_id=0  sample_time=0.000500
  Pelvis Right Reed Switch PDO Receive : xpcethercatlib/EtherCAT PDO Receive  Priority=2  sig_name=Pelvis Medulla.Misc Inputs.Right Reed Switch State  sig_offset=1825  sig_type=boolean  type_size=1  sig_dim=1  device_id=0  sample_time=0.000500
  Piezo State Bus Selector : BusSelector  OutputSignals=pelvisMedulla.miscOutputs.piezoState
  Piezo State PDO Transmit : xpcethercatlib/EtherCAT PDO Transmit   Priority=3  sig_name=Pelvis Medulla.Misc Outputs.Piezo State  sig_offset=817  sig_type=boolean  type_size=1  sig_dim=1  device_id=0  sample_time=0.000500
  Piezo Tone Bus Selector : BusSelector  OutputSignals=pelvisMedulla.miscOutputs.piezoTone
  Piezo Tone PDO Transmit : xpcethercatlib/EtherCAT PDO Transmit   Priority=3  sig_name=Pelvis Medulla.Misc Outputs.Piezo Tone  sig_offset=824  sig_type=uint8  type_size=8  sig_dim=1  device_id=0  sample_time=0.000500
  Safe Torque Off Bus Selector : BusSelector  OutputSignals=pelvisMedulla.miscOutputs.sto
  Safe Torque Off PDO Transmit : xpcethercatlib/EtherCAT PDO Transmit   Priority=3  sig_name=Pelvis Medulla.Misc Outputs.Medulla STO  sig_offset=816  sig_type=boolean  type_size=1  sig_dim=1  device_id=0  sample_time=0.000500
  VTM Temperature PDO Receive : xpcethercatlib/EtherCAT PDO Receive  Priority=2  sig_name=Pelvis Medulla.Misc Inputs.VTM Temperature  sig_offset=1832  sig_type=int16  type_size=16  sig_dim=1  device_id=0  sample_time=0.000500
  Outport : Outport
  wires:
  Misc Inputs Bus Assignment/1 -> Outport/1
  Piezo Tone Bus Selector/1 -> Piezo Tone PDO Transmit/1  "<piezoTone>"
  Piezo State Bus Selector/1 -> Piezo State PDO Transmit/1  "<piezoState>"
  Safe Torque Off Bus Selector/1 -> Safe Torque Off PDO Transmit/1  "<sto>"
  Inport/1 -> Misc Inputs Bus Assignment/1, Piezo State Bus Selector/1, Safe Torque Off Bus Selector/1, Piezo Tone Bus Selector/1
  ADC to Celcius MATLAB Function/1(C) -> Misc Inputs Bus Assignment/5
  Bleeder Triggered PDO Receive/1 -> Misc Inputs Bus Assignment/4
  Pelvis Right Reed Switch PDO Receive/1 -> Misc Inputs Bus Assignment/3
  Pelvis Left Reed Switch PDO Receive/1 -> Misc Inputs Bus Assignment/2
  VTM Temperature PDO Receive/1 -> ADC to Celcius MATLAB Function/1(adcValue)

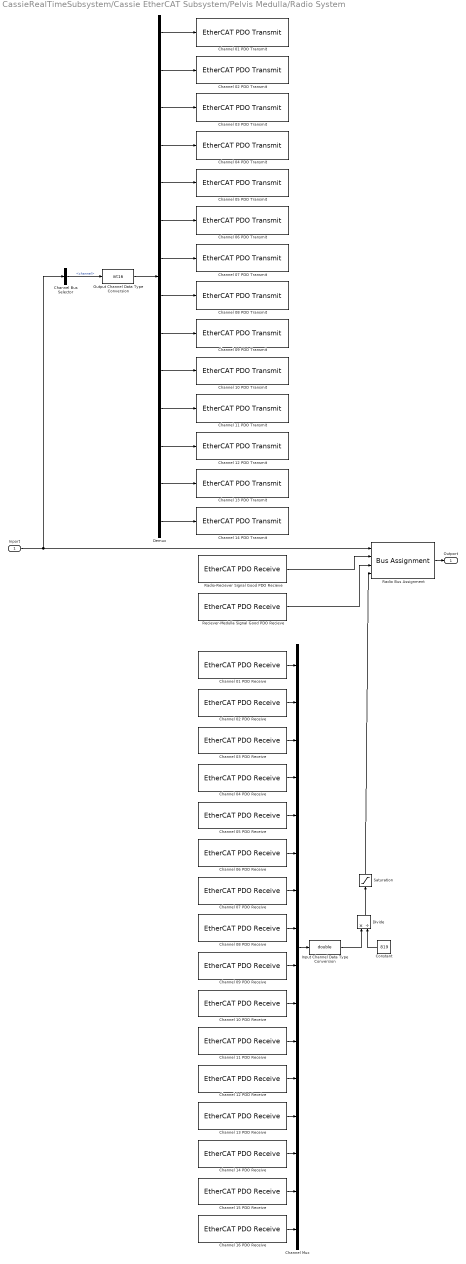
== system CassieRealTimeSubsystem/Cassie EtherCAT Subsystem/Pelvis Medulla/Radio System ==
  Inport : Inport
  Channel Bus Selector : BusSelector  OutputSignals=pelvisMedulla.radioOutputs.channel
  Channel Mux : Mux  Inputs=16
  Channel 01 PDO Receive : xpcethercatlib/EtherCAT PDO Receive  Priority=2  sig_name=Pelvis Medulla.Radio Inputs.Channel 01  sig_offset=616  sig_type=int16  type_size=16  sig_dim=1  device_id=0  sample_time=0.000500
  Channel 01 PDO Transmit : xpcethercatlib/EtherCAT PDO Transmit   Priority=3  sig_name=Pelvis Medulla.Radio Outputs.Channel 01  sig_offset=592  sig_type=int16  type_size=16  sig_dim=1  device_id=0  sample_time=0.000500
  Channel 02 PDO Receive : xpcethercatlib/EtherCAT PDO Receive  Priority=2  sig_name=Pelvis Medulla.Radio Inputs.Channel 02  sig_offset=632  sig_type=int16  type_size=16  sig_dim=1  device_id=0  sample_time=0.000500
  Channel 02 PDO Transmit : xpcethercatlib/EtherCAT PDO Transmit   Priority=3  sig_name=Pelvis Medulla.Radio Outputs.Channel 02  sig_offset=608  sig_type=int16  type_size=16  sig_dim=1  device_id=0  sample_time=0.000500
  Channel 03 PDO Receive : xpcethercatlib/EtherCAT PDO Receive  Priority=2  sig_name=Pelvis Medulla.Radio Inputs.Channel 03  sig_offset=648  sig_type=int16  type_size=16  sig_dim=1  device_id=0  sample_time=0.000500
  Channel 03 PDO Transmit : xpcethercatlib/EtherCAT PDO Transmit   Priority=3  sig_name=Pelvis Medulla.Radio Outputs.Channel 03  sig_offset=624  sig_type=int16  type_size=16  sig_dim=1  device_id=0  sample_time=0.000500
  Channel 04 PDO Receive : xpcethercatlib/EtherCAT PDO Receive  Priority=2  sig_name=Pelvis Medulla.Radio Inputs.Channel 04  sig_offset=664  sig_type=int16  type_size=16  sig_dim=1  device_id=0  sample_time=0.000500
  Channel 04 PDO Transmit : xpcethercatlib/EtherCAT PDO Transmit   Priority=3  sig_name=Pelvis Medulla.Radio Outputs.Channel 04  sig_offset=640  sig_type=int16  type_size=16  sig_dim=1  device_id=0  sample_time=0.000500
  Channel 05 PDO Receive : xpcethercatlib/EtherCAT PDO Receive  Priority=2  sig_name=Pelvis Medulla.Radio Inputs.Channel 05  sig_offset=680  sig_type=int16  type_size=16  sig_dim=1  device_id=0  sample_time=0.000500
  Channel 05 PDO Transmit : xpcethercatlib/EtherCAT PDO Transmit   Priority=3  sig_name=Pelvis Medulla.Radio Outputs.Channel 05  sig_offset=656  sig_type=int16  type_size=16  sig_dim=1  device_id=0  sample_time=0.000500
  Channel 06 PDO Receive : xpcethercatlib/EtherCAT PDO Receive  Priority=2  sig_name=Pelvis Medulla.Radio Inputs.Channel 06  sig_offset=696  sig_type=int16  type_size=16  sig_dim=1  device_id=0  sample_time=0.000500
  Channel 06 PDO Transmit : xpcethercatlib/EtherCAT PDO Transmit   Priority=3  sig_name=Pelvis Medulla.Radio Outputs.Channel 06  sig_offset=672  sig_type=int16  type_size=16  sig_dim=1  device_id=0  sample_time=0.000500
  Channel 07 PDO Receive : xpcethercatlib/EtherCAT PDO Receive  Priority=2  sig_name=Pelvis Medulla.Radio Inputs.Channel 07  sig_offset=712  sig_type=int16  type_size=16  sig_dim=1  device_id=0  sample_time=0.000500
  Channel 07 PDO Transmit : xpcethercatlib/EtherCAT PDO Transmit   Priority=3  sig_name=Pelvis Medulla.Radio Outputs.Channel 07  sig_offset=688  sig_type=int16  type_size=16  sig_dim=1  device_id=0  sample_time=0.000500
  Channel 08 PDO Receive : xpcethercatlib/EtherCAT PDO Receive  Priority=2  sig_name=Pelvis Medulla.Radio Inputs.Channel 08  sig_offset=728  sig_type=int16  type_size=16  sig_dim=1  device_id=0  sample_time=0.000500
  Channel 08 PDO Transmit : xpcethercatlib/EtherCAT PDO Transmit   Priority=3  sig_name=Pelvis Medulla.Radio Outputs.Channel 08  sig_offset=704  sig_type=int16  type_size=16  sig_dim=1  device_id=0  sample_time=0.000500
  Channel 09 PDO Receive : xpcethercatlib/EtherCAT PDO Receive  Priority=2  sig_name=Pelvis Medulla.Radio Inputs.Channel 09  sig_offset=744  sig_type=int16  type_size=16  sig_dim=1  device_id=0  sample_time=0.000500
  Channel 09 PDO Transmit : xpcethercatlib/EtherCAT PDO Transmit   Priority=3  sig_name=Pelvis Medulla.Radio Outputs.Channel 09  sig_offset=720  sig_type=int16  type_size=16  sig_dim=1  device_id=0  sample_time=0.000500
  Channel 10 PDO Receive : xpcethercatlib/EtherCAT PDO Receive  Priority=2  sig_name=Pelvis Medulla.Radio Inputs.Channel 10  sig_offset=760  sig_type=int16  type_size=16  sig_dim=1  device_id=0  sample_time=0.000500
  Channel 10 PDO Transmit : xpcethercatlib/EtherCAT PDO Transmit   Priority=3  sig_name=Pelvis Medulla.Radio Outputs.Channel 10  sig_offset=736  sig_type=int16  type_size=16  sig_dim=1  device_id=0  sample_time=0.000500
  Channel 11 PDO Receive : xpcethercatlib/EtherCAT PDO Receive  Priority=2  sig_name=Pelvis Medulla.Radio Inputs.Channel 11  sig_offset=776  sig_type=int16  type_size=16  sig_dim=1  device_id=0  sample_time=0.000500
  Channel 11 PDO Transmit : xpcethercatlib/EtherCAT PDO Transmit   Priority=3  sig_name=Pelvis Medulla.Radio Outputs.Channel 11  sig_offset=752  sig_type=int16  type_size=16  sig_dim=1  device_id=0  sample_time=0.000500
  Channel 12 PDO Receive : xpcethercatlib/EtherCAT PDO Receive  Priority=2  sig_name=Pelvis Medulla.Radio Inputs.Channel 12  sig_offset=792  sig_type=int16  type_size=16  sig_dim=1  device_id=0  sample_time=0.000500
  Channel 12 PDO Transmit : xpcethercatlib/EtherCAT PDO Transmit   Priority=3  sig_name=Pelvis Medulla.Radio Outputs.Channel 12  sig_offset=768  sig_type=int16  type_size=16  sig_dim=1  device_id=0  sample_time=0.000500
  Channel 13 PDO Receive : xpcethercatlib/EtherCAT PDO Receive  Priority=2  sig_name=Pelvis Medulla.Radio Inputs.Channel 13  sig_offset=808  sig_type=int16  type_size=16  sig_dim=1  device_id=0  sample_time=0.000500
  Channel 13 PDO Transmit : xpcethercatlib/EtherCAT PDO Transmit   Priority=3  sig_name=Pelvis Medulla.Radio Outputs.Channel 13  sig_offset=784  sig_type=int16  type_size=16  sig_dim=1  device_id=0  sample_time=0.000500
  Channel 14 PDO Receive : xpcethercatlib/EtherCAT PDO Receive  Priority=2  sig_name=Pelvis Medulla.Radio Inputs.Channel 14  sig_offset=824  sig_type=int16  type_size=16  sig_dim=1  device_id=0  sample_time=0.000500
  Channel 14 PDO Transmit : xpcethercatlib/EtherCAT PDO Transmit   Priority=3  sig_name=Pelvis Medulla.Radio Outputs.Channel 14  sig_offset=800  sig_type=int16  type_size=16  sig_dim=1  device_id=0  sample_time=0.000500
  Channel 15 PDO Receive : xpcethercatlib/EtherCAT PDO Receive  Priority=2  sig_name=Pelvis Medulla.Radio Inputs.Channel 15  sig_offset=840  sig_type=int16  type_size=16  sig_dim=1  device_id=0  sample_time=0.000500
  Channel 16 PDO Receive : xpcethercatlib/EtherCAT PDO Receive  Priority=2  sig_name=Pelvis Medulla.Radio Inputs.Channel 16  sig_offset=856  sig_type=int16  type_size=16  sig_dim=1  device_id=0  sample_time=0.000500
  Constant : Constant  Value=819
  Demux : Demux  Outputs=14
  Divide : Product  Inputs=*/
  Input Channel Data Type Conversion : DataTypeConversion  OutDataTypeStr=double
  Output Channel Data Type Conversion : DataTypeConversion  OutDataTypeStr=int16
  Radio Bus Assignment : BusAssignment  AssignedSignals=pelvisMedulla.radioInputs.radioReceiverSignalGood,pelvisMedulla.radioInputs.receiverMedullaSignalGood,pelvisMedulla.radioInputs.channel
  Radio-Reciever Signal Good PDO Recieve : xpcethercatlib/EtherCAT PDO Receive  Priority=2  sig_name=Pelvis Medulla.Radio Inputs.Radio-Receiver Signal Good  sig_offset=872  sig_type=boolean  type_size=1  sig_dim=1  device_id=0  sample_time=0.000500
  Reciever-Medulla Signal Good PDO Recieve : xpcethercatlib/EtherCAT PDO Receive  Priority=2  sig_name=Pelvis Medulla.Radio Inputs.Receiver-Medulla Signal Good  sig_offset=873  sig_type=boolean  type_size=1  sig_dim=1  device_id=0  sample_time=0.000500
  Saturation : Saturate  UpperLimit=1  LowerLimit=-1
  Outport : Outport
  wires:
  Radio Bus Assignment/1 -> Outport/1
  Channel 01 PDO Receive/1 -> Channel Mux/1
  Channel 02 PDO Receive/1 -> Channel Mux/2
  Channel 16 PDO Receive/1 -> Channel Mux/16
  Channel 15 PDO Receive/1 -> Channel Mux/15
  Channel 14 PDO Receive/1 -> Channel Mux/14
  Channel 13 PDO Receive/1 -> Channel Mux/13
  Channel 12 PDO Receive/1 -> Channel Mux/12
  Channel 11 PDO Receive/1 -> Channel Mux/11
  Channel 10 PDO Receive/1 -> Channel Mux/10
  Channel 09 PDO Receive/1 -> Channel Mux/9
  Channel 08 PDO Receive/1 -> Channel Mux/8
  Channel 06 PDO Receive/1 -> Channel Mux/6
  Channel 07 PDO Receive/1 -> Channel Mux/7
  Channel 03 PDO Receive/1 -> Channel Mux/3
  Channel 04 PDO Receive/1 -> Channel Mux/4
  Channel 05 PDO Receive/1 -> Channel Mux/5
  Channel Mux/1 -> Input Channel Data Type Conversion/1
  Reciever-Medulla Signal Good PDO Recieve/1 -> Radio Bus Assignment/3
  Radio-Reciever Signal Good PDO Recieve/1 -> Radio Bus Assignment/2
  Channel Bus Selector/1 -> Output Channel Data Type Conversion/1  "<channel>"
  Inport/1 -> Channel Bus Selector/1, Radio Bus Assignment/1
  Demux/1 -> Channel 01 PDO Transmit/1
  Demux/14 -> Channel 14 PDO Transmit/1
  Demux/2 -> Channel 02 PDO Transmit/1
  Demux/3 -> Channel 03 PDO Transmit/1
  Demux/4 -> Channel 04 PDO Transmit/1
  Demux/5 -> Channel 05 PDO Transmit/1
  Demux/6 -> Channel 06 PDO Transmit/1
  Demux/7 -> Channel 07 PDO Transmit/1
  Demux/8 -> Channel 08 PDO Transmit/1
  Demux/9 -> Channel 09 PDO Transmit/1
  Demux/10 -> Channel 10 PDO Transmit/1
  Demux/11 -> Channel 11 PDO Transmit/1
  Demux/12 -> Channel 12 PDO Transmit/1
  Demux/13 -> Channel 13 PDO Transmit/1
  Output Channel Data Type Conversion/1 -> Demux/1
  Input Channel Data Type Conversion/1 -> Divide/1
  Constant/1 -> Divide/2
  Divide/1 -> Saturation/1
  Saturation/1 -> Radio Bus Assignment/4
